simulink model "PR_planningsim_2joint"  (R2024a)
settings: Solver=ode45  StartTime=0.0  StopTime=stoptime
undefined symbols (not defined in the file): amp_factor, arm_radius, arm_radius_previus, begintime, controlactivate, damping_coeff, I_est, ifreskicking, ifreslosetrack, ifresnoise, ifrobotkicking, ifrobotnoise, ini_theta_p, ini_thetadot_p, pendepth, penlength, penposx, penposz, penrho, penwidth, rc, res_kick_height, res_kick_period, res_kick_start, res_losetrack_period, res_losetrack_start, res_noise_seed, res_noise_variance, robot_kick_height, robot_kick_period, robot_kick_start, robot_noise_seed, robot_noise_variance, robot_pendepth, robot_penlength, robot_penwidth, robot_pulse_freq, robot_pulse_hight, robot_pulse_period, robot_pulse_start, robot_sphere_mass, samplingrate, sphere_mass, sphere_radius, spring_position_scale, switch_threshold, torquelim, Win, X, Y, Z
libraries: sm_lib x25, nesl_utility x11, dspindex x5
(part 1 of 2)
settings Model: Creator=fy264  LastModifiedBy=fy264
settings OptimizationCC: ReuseModelBlockBuffer=off
settings DebuggingCC: AlgebraicLoopMsg=none  ArtificialAlgebraicLoopMsg=none
settings RTWCC: GPUComputeCapability=3.5
settings ExplorerConfigSet: InternalSimMechanicsExplorerSettings="<ExplorerConfiguration><canonicalview>default</canonicalview><AnimationSetting><BasePlaybackSpeed>1.0</BasePlaybackSpeed><PlaybackSpeedFactor>1.0</PlaybackSpeedFactor></AnimationSetting><TilePanel><TileInfo><Tiles Columns=\"1\" Count=\"1\" Rows=\"1\"><Column Weight=\"1\"/><Row Weight=\"1\"/><Tile Height=\"1\" Width=\"1\" X=\"0\" Y=\"0\"/></Tiles></TileInfo><SceneInfo><SceneViewer><BGColor><R>1</R><G>1</G><B>1</B></BGColor><Camera><DoPerspective>off</DoPerspective><Position><X>0.124591896750282635</X><Y>-1</Y><Z>0.0418966536850959165</Z></Position><Center><X>0.124591896750282635</X><Y>-3.46944695195361419e-18</Y><Z>0.0418966536850959165</Z></Center><Up><X>0</X><Y>-0</Y><Z>1</Z></Up><ViewLimDist>1</ViewLimDist><YLim>0.484627616003313111</YLim><XLim>0.343227538516062136</XLim></Camera></SceneViewer></SceneInfo></TilePanel><MechEditorPanel><Cameras/><GfxPanelCameraMap/><VideoCreator><PlaybackSpeedRatio>1.0</PlaybackSpeedRatio><FrameRate>30</FrameRate><VideoFormat>Motion JPEG AVI</VideoFormat><FrameSize>auto</FrameSize></VideoCreator></MechEditorPanel></ExplorerConfiguration>"

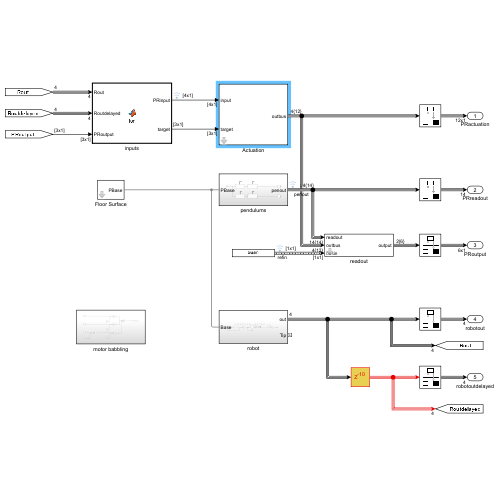
[thumbnail: Simulink's stored preview of the top-level diagram]
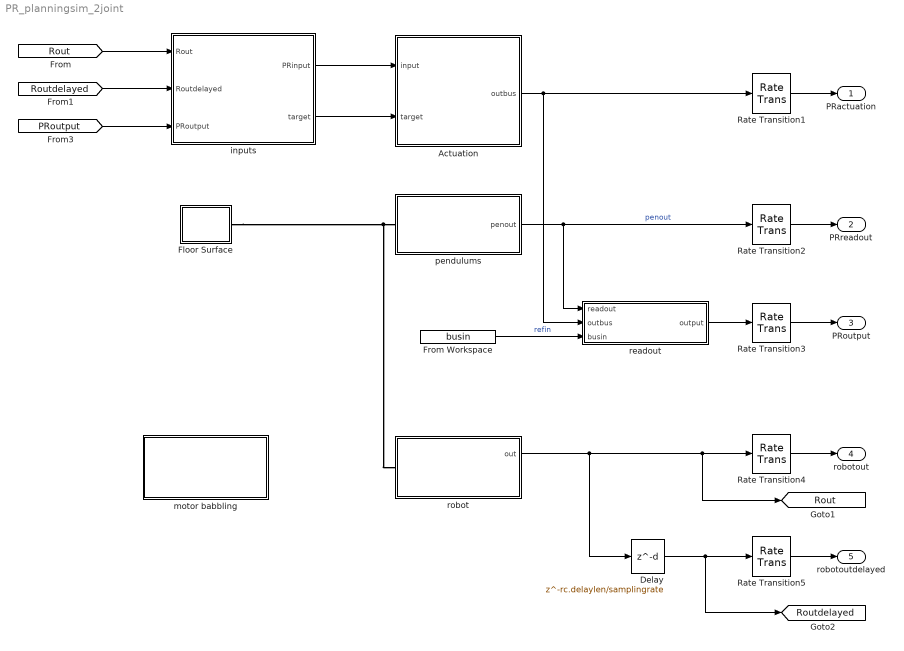
== system PR_planningsim_2joint ==
  Actuation : Subsystem  mask{xnorm=rc.xnorm}
  Delay : Delay  DelayLength=rc.delaylen/samplingrate  InitialCondition=0
  Floor Surface : Subsystem  mask{length=0.5, width=0.5}
      mask prompts: length "grid length [m]"; width "grid width [m]"
  From Workspace : FromWorkspace  VariableName=busin  OutDataTypeStr=Bus: SinusoidBus  OutputAfterFinalValue=Holding final value
  Rate Transition{1..5} (5 alike) : RateTransition  OutPortSampleTime=samplingrate
  inputs : MATLAB Function  TreatAsAtomicUnit=on
  motor babbling : Subsystem
  pendulums : Subsystem
  readout : Subsystem  mask{Woutmat=rc.Woutmat}
  robot : Subsystem
  PRactuation : Outport
  PRreadout : Outport  Port=2
  PRoutput : Outport  Port=3
  robotout : Outport  Port=4
  robotoutdelayed : Outport  Port=5
  tag scope: Rout=global, Routdelayed=global
  wires:
  Actuation/1(outbus) -> readout/2(outbus), Rate Transition1/1
  Rate Transition1/1 -> PRactuation/1
  pendulums/1(penout) -> readout/1(readout), Rate Transition2/1  "penout"
  Rate Transition2/1 -> PRreadout/1
  readout/1(output) -> Rate Transition3/1
  Rate Transition3/1 -> PRoutput/1
  Rate Transition4/1 -> robotout/1
  inputs/1(PRinput) -> Actuation/1(input)
  [Rout] -> inputs/1(Rout)
  Rate Transition5/1 -> robotoutdelayed/1
  robot/1(out) -> Delay/1, Rate Transition4/1, [Rout]
  Delay/1 -> [Routdelayed], Rate Transition5/1
  [Routdelayed] -> inputs/2(Routdelayed)
  inputs/2(target) -> Actuation/2(target)
  [PRoutput] -> inputs/3(PRoutput)
  From Workspace/1 -> readout/3(busin)  "refin"
  connections:
  Floor Surface/RConn1 -- robot/LConn1 -- pendulums/LConn1

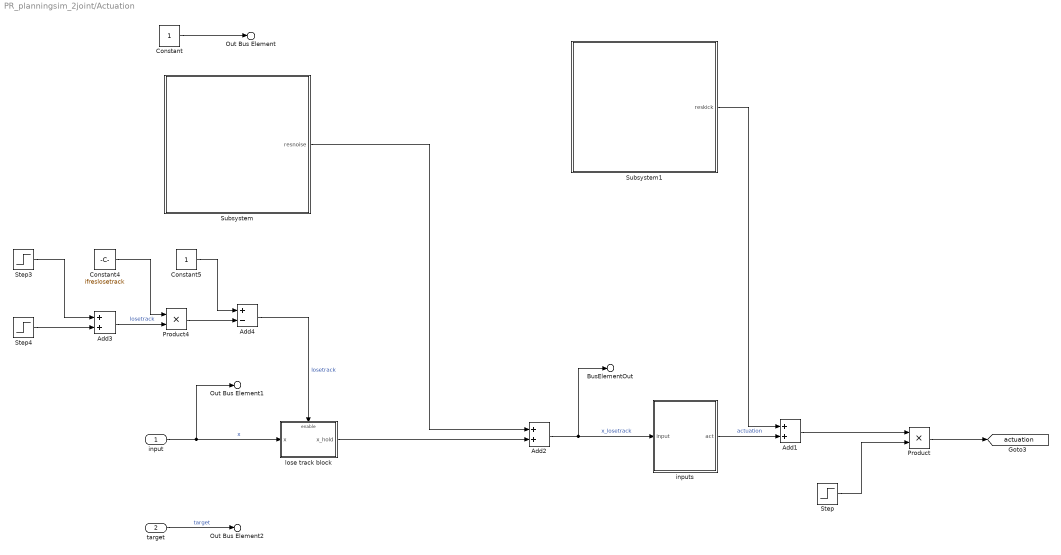
== system PR_planningsim_2joint/Actuation ==
  input : Inport
  target : Inport  Port=2
  Add1 : Sum
  Add2 : Sum
  Add3 : Sum
  Add4 : Sum  Inputs=+-
  Constant : Constant
  Constant4 : Constant  Value=ifreslosetrack
  Constant5 : Constant
  Product : Product
  Product4 : Product
  Step : Step  Time=begintime  SampleTime=0
  Step3 : Step  Time=res_losetrack_start  SampleTime=0
  Step4 : Step  Time=res_losetrack_start+res_losetrack_period  After=-1  SampleTime=0
  Subsystem : Subsystem
  Subsystem1 : Subsystem
  inputs : MATLAB Function  TreatAsAtomicUnit=on
  lose track block : Subsystem
  Out Bus Element : Outport  PortName=outbus  Element=const
  Out Bus Element1 : Outport  PortName=outbus  Element=x
  Out Bus Element2 : Outport  PortName=outbus  Element=target
  BusElementOut : Outport  PortName=outbus  Element=x_lost
  tag scope: actuation=global
  wires:
  input/1 -> Out Bus Element1/1, lose track block/1(x)  "x"
  Constant/1 -> Out Bus Element/1
  target/1 -> Out Bus Element2/1  "target"
  inputs/1(act) -> Add1/2  "actuation"
  Step/1 -> Product/2
  Step4/1 -> Add3/2
  Add3/1 -> Product4/2  "losetrack"
  Step3/1 -> Add3/1
  Constant4/1 -> Product4/1
  Constant5/1 -> Add4/1
  Product4/1 -> Add4/2
  Add4/1 -> lose track block/Enable  "losetrack"
  Product/1 -> [actuation]
  Add2/1 -> inputs/1(input), BusElementOut/1  "x_losetrack"
  Subsystem/1(resnoise) -> Add2/1
  lose track block/1(x_hold) -> Add2/2
  Add1/1 -> Product/1
  Subsystem1/1(reskick) -> Add1/1

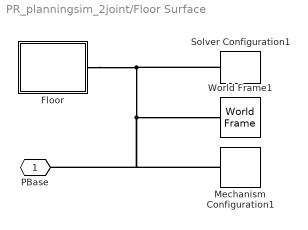
== system PR_planningsim_2joint/Floor Surface ==
  Floor : Subsystem
  Mechanism Configuration1 : sm_lib/Utilities/Mechanism Configuration  UniformGravity=Constant  GravityVector=[0 0 -9.80665]  GravityVectorUnits=m/s^2  LinearizationDelta=0.001  JointModeTransitionNonlinearIterations=2
  Solver Configuration1 : nesl_utility/Solver Configuration  PhysicalDomain=network_engine_domain  SubClassName=solver  LeftPortType=input  RightPortType=generic  Tones=[]  Harmonics=[]  SimulateNoise=off  Profile=off  UseLocalSampling=off  EnableSwitchedLinearOptims=on  FrequencyDomain=off  UseCCode=off  RelTol=0.001  AbsTol=1e-06  MinStep=1e-09  ToWorkspace=off  RevertToSquareIcSolve=off  NumHomotopyIterations=100  PhasorMode=off  PhasorModeNumHarmonics=1  ConsistencySolver=NEWTON_FTOL  IndexReductionMethod=DerivativeReplacement  DoDC=off  ResidualTolerance=1e-09  ConsistencyTolSource=GLOBAL  ConsistencyAbsTol=0.001  ConsistencyRelTol=0.001  ConsistencyTolFactor=0.001  UseLocalSolver=off  LocalSolverChoice=NE_BACKWARD_EULER_ADVANCER  ResolveIndetEquations=on  FunctionEvalNumThread=1  LocalSolverSampleTime=0.0002  DoFixedCost=off  MaxNonlinIter=10  MaxModeIter=2  ComputeImpulses=off  ImpulseIterations=2  LinearAlgebra=Sparse  LinearAlgebraNumThread=0  EquationFormulation=NE_TIME_EF  DelaysMemoryBudget=1024  AutomaticFiltering=off  FilteringTimeConstant=0.001  PartitionStorageMethod=AS_NEEDED  PartitionMemoryBudget=1024  PartitionMethod=FAST  MultibodyUseLocalSolver=off  MultibodyLocalSolverChoice=ODE1  MultibodyLocalSolverSampleTime=0.001
  World Frame1 : sm_lib/Frames and Transforms/World Frame
  PBase : PMIOPort  Side=Right
  connections:
  Floor/RConn1 -- PBase/RConn1 -- Mechanism Configuration1/RConn1 -- World Frame1/RConn1 -- Solver Configuration1/RConn1

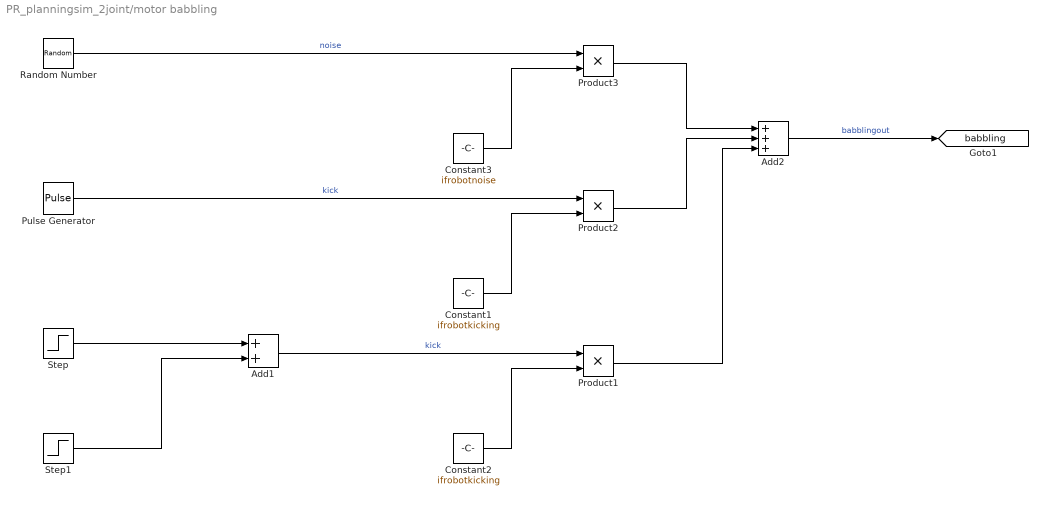
== system PR_planningsim_2joint/motor babbling ==
  Add1 : Sum
  Add2 : Sum  Inputs=+++
  Constant1 : Constant  Value=ifrobotkicking
  Constant2 : Constant  Value=ifrobotkicking
  Constant3 : Constant  Value=ifrobotnoise
  Product1 : Product
  Product2 : Product
  Product3 : Product
  Pulse Generator : DiscretePulseGenerator  PulseType=Time based  Amplitude=robot_pulse_hight  Period=1/robot_pulse_freq  PulseWidth=robot_pulse_period*robot_pulse_freq  PhaseDelay=robot_pulse_start
  Random Number : RandomNumber  Variance=robot_noise_variance  Seed=robot_noise_seed  SampleTime=samplingrate
  Step : Step  Time=robot_kick_start  After=robot_kick_height  SampleTime=0
  Step1 : Step  Time=robot_kick_start+robot_kick_period  After=-robot_kick_height  SampleTime=0
  tag scope: babbling=global
  wires:
  Step/1 -> Add1/1
  Step1/1 -> Add1/2
  Constant2/1 -> Product1/2
  Add2/1 -> [babbling]  "babblingout"
  Add1/1 -> Product1/1  "kick"
  Constant1/1 -> Product2/2
  Pulse Generator/1 -> Product2/1  "kick"
  Constant3/1 -> Product3/2
  Product3/1 -> Add2/1
  Product2/1 -> Add2/2
  Product1/1 -> Add2/3
  Random Number/1 -> Product3/1  "noise"

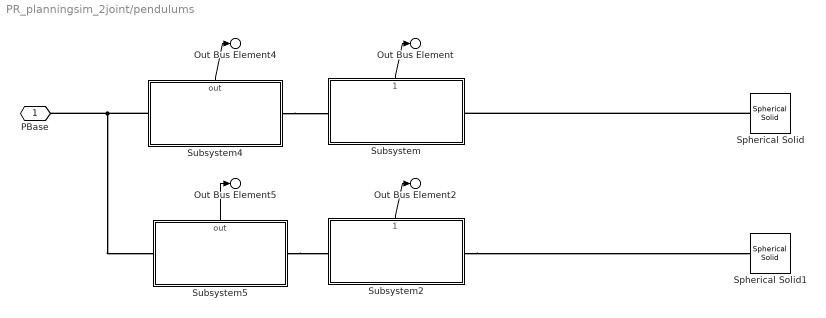
== system PR_planningsim_2joint/pendulums ==
  Spherical Solid : sm_lib/Body Elements/Spherical Solid  SphereRadius=sphere_radius(1, 3)  SphereRadiusUnits=m  ExportEntireGeometry=off  InertiaType=CalculateFromGeometry  BasedOnType=Mass  Density=1000  DensityUnits=kg/m^3  Mass=sphere_mass(1, 1)  MassUnits=kg  CenterOfMass=[0 0 0]  CenterOfMassUnits=m  MomentsOfInertia=[1 1 1]  MomentsOfInertiaUnits=kg*m^2  ProductsOfInertia=[0 0 0]  ProductsOfInertiaUnits=kg*m^2  GraphicType=FromGeometry  MarkerShape=Sphere  MarkerSize=10  GraphicVisPropType=SimpleVisualProperties  GraphicDiffuseColor=[0.6 0.6 0.6]  GraphicOpacity=1.0  GraphicSpecularColor=[0.5 0.5 0.5 1.0]  GraphicAmbientColor=[0.15 0.15 0.15 1.0]  GraphicEmissiveColor=[0.0 0.0 0.0 1.0]  GraphicShininess=75  DoExposeReferenceFrame=on  SerializedFrames=<Frames><Frame><Id>Frame1</Id><Value><Name>F1</Name><Origin><Source>ReferenceFrame</Source><FeatureName></FeatureName></Origin><PrimaryAxis><DefinedDirection>+Z</DefinedDirection><Source>ReferenceFrame</Source><SourceDirection>+Z</SourceDirection><FeatureName></FeatureName></PrimaryAxis><SecondaryAxis><DefinedDirection>+X</DefinedDirection><Source>ReferenceFrame</Source><SourceDirection>+X</SourceDirection><FeatureName></FeatureName></SecondaryAxis></Value></Frame></Frames>
  Spherical Solid1 : sm_lib/Body Elements/Spherical Solid  SphereRadius=sphere_radius(2, 3)  SphereRadiusUnits=m  ExportEntireGeometry=off  InertiaType=CalculateFromGeometry  BasedOnType=Mass  Density=1000  DensityUnits=kg/m^3  Mass=sphere_mass(1, 1)  MassUnits=kg  CenterOfMass=[0 0 0]  CenterOfMassUnits=m  MomentsOfInertia=[1 1 1]  MomentsOfInertiaUnits=kg*m^2  ProductsOfInertia=[0 0 0]  ProductsOfInertiaUnits=kg*m^2  GraphicType=FromGeometry  MarkerShape=Sphere  MarkerSize=10  GraphicVisPropType=SimpleVisualProperties  GraphicDiffuseColor=[0.6 0.6 0.6]  GraphicOpacity=1.0  GraphicSpecularColor=[0.5 0.5 0.5 1.0]  GraphicAmbientColor=[0.15 0.15 0.15 1.0]  GraphicEmissiveColor=[0.0 0.0 0.0 1.0]  GraphicShininess=75  DoExposeReferenceFrame=on  SerializedFrames=<Frames><Frame><Id>Frame1</Id><Value><Name>F1</Name><Origin><Source>ReferenceFrame</Source><FeatureName></FeatureName></Origin><PrimaryAxis><DefinedDirection>+Z</DefinedDirection><Source>ReferenceFrame</Source><SourceDirection>+Z</SourceDirection><FeatureName></FeatureName></PrimaryAxis><SecondaryAxis><DefinedDirection>+X</DefinedDirection><Source>ReferenceFrame</Source><SourceDirection>+X</SourceDirection><FeatureName></FeatureName></SecondaryAxis></Value></Frame></Frames>
  Subsystem : Subsystem  ReferencedSubsystem=pendulum_refsin  pendulum_label=[1 2]
      settings: PortSchema="{\"entries\":[{\"content\":{\"sides\":[{\"content\":{\"connectorIds\":[\"LConn1\"]},\"type\":\"ConnectorPlacement.EquallySpacedRectSide\",\"uuid\":\"2e961fb3-335c-4cac-865d-869b1ba40a20\"},{\"content\":{\"connectorIds\":[\"RConn1\"],\"side\":\"RIGHT\"},\"type\":\"ConnectorPlacement.EquallySpacedRectSide\",\"uuid\":\"69169429-8ae9-43d1-9e87-82c377e9f397\"},{\"content\":{\"connectorIds\":[\"Out1\"],\"side\":\"TOP\"},\"type\":\"ConnectorPlacement.EquallySpacedRectSide\",\"uuid\":\"d66a7b83-282b-4030-adef-01b228f0b3fc\"}]},\"type\":\"ConnectorPlacement.EquallySpacedConnector\",\"uuid\":\"3d306e9c-76f1-4223-9644-f2ea4df9a3d0\"}],\"packageUris\":[\"http://schema.mathworks.com/mf0/Connector/R2020b\"],\"version\":\"1.0\"}"
  Subsystem2 : Subsystem  ReferencedSubsystem=pendulum_refsin  pendulum_label=[2 2]
      settings: PortSchema="{\"entries\":[{\"content\":{\"sides\":[{\"content\":{\"connectorIds\":[\"LConn1\"]},\"type\":\"ConnectorPlacement.EquallySpacedRectSide\",\"uuid\":\"2e961fb3-335c-4cac-865d-869b1ba40a20\"},{\"content\":{\"connectorIds\":[\"RConn1\"],\"side\":\"RIGHT\"},\"type\":\"ConnectorPlacement.EquallySpacedRectSide\",\"uuid\":\"69169429-8ae9-43d1-9e87-82c377e9f397\"},{\"content\":{\"connectorIds\":[\"Out1\"],\"side\":\"TOP\"},\"type\":\"ConnectorPlacement.EquallySpacedRectSide\",\"uuid\":\"d66a7b83-282b-4030-adef-01b228f0b3fc\"}]},\"type\":\"ConnectorPlacement.EquallySpacedConnector\",\"uuid\":\"3d306e9c-76f1-4223-9644-f2ea4df9a3d0\"}],\"packageUris\":[\"http://schema.mathworks.com/mf0/Connector/R2020b\"],\"version\":\"1.0\"}"
  Subsystem4 : Subsystem  mask{pendulum_label=[1 1]}
      settings: PortSchema="{\"entries\":[{\"content\":{\"sides\":[{\"content\":{\"connectorIds\":[\"LConn1\"]},\"type\":\"ConnectorPlacement.EquallySpacedRectSide\",\"uuid\":\"2e961fb3-335c-4cac-865d-869b1ba40a20\"},{\"content\":{\"connectorIds\":[\"RConn1\"],\"side\":\"RIGHT\"},\"type\":\"ConnectorPlacement.EquallySpacedRectSide\",\"uuid\":\"69169429-8ae9-43d1-9e87-82c377e9f397\"},{\"content\":{\"connectorIds\":[\"Out1\"],\"side\":\"TOP\"},\"type\":\"ConnectorPlacement.EquallySpacedRectSide\",\"uuid\":\"d66a7b83-282b-4030-adef-01b228f0b3fc\"}]},\"type\":\"ConnectorPlacement.EquallySpacedConnector\",\"uuid\":\"3d306e9c-76f1-4223-9644-f2ea4df9a3d0\"}],\"packageUris\":[\"http://schema.mathworks.com/mf0/Connector/R2020b\"],\"version\":\"1.0\"}"
  Subsystem5 : Subsystem  mask{pendulum_label=[2 1]}
      settings: PortSchema="{\"entries\":[{\"content\":{\"sides\":[{\"content\":{\"connectorIds\":[\"LConn1\"]},\"type\":\"ConnectorPlacement.EquallySpacedRectSide\",\"uuid\":\"2e961fb3-335c-4cac-865d-869b1ba40a20\"},{\"content\":{\"connectorIds\":[\"RConn1\"],\"side\":\"RIGHT\"},\"type\":\"ConnectorPlacement.EquallySpacedRectSide\",\"uuid\":\"69169429-8ae9-43d1-9e87-82c377e9f397\"},{\"content\":{\"connectorIds\":[\"Out1\"],\"side\":\"TOP\"},\"type\":\"ConnectorPlacement.EquallySpacedRectSide\",\"uuid\":\"d66a7b83-282b-4030-adef-01b228f0b3fc\"}]},\"type\":\"ConnectorPlacement.EquallySpacedConnector\",\"uuid\":\"3d306e9c-76f1-4223-9644-f2ea4df9a3d0\"}],\"packageUris\":[\"http://schema.mathworks.com/mf0/Connector/R2020b\"],\"version\":\"1.0\"}"
  PBase : PMIOPort  Side=Left
  Out Bus Element4 : Outport  PortName=penout  Element=pendulum_1_0
  Out Bus Element : Outport  PortName=penout  Element=pendulum_1_1
  Out Bus Element5 : Outport  PortName=penout  Element=pendulum_2_0
  Out Bus Element2 : Outport  PortName=penout  Element=pendulum_2_1
  wires:
  Subsystem2/1 -> Out Bus Element2/1
  Subsystem/1 -> Out Bus Element/1
  Subsystem4/1(out) -> Out Bus Element4/1
  Subsystem5/1(out) -> Out Bus Element5/1
  connections:
  Spherical Solid/LConn1 -- Subsystem/RConn1
  Subsystem2/RConn1 -- Spherical Solid1/LConn1
  Subsystem4/RConn1 -- Subsystem/LConn1
  Subsystem4/LConn1 -- Subsystem5/LConn1 -- PBase/RConn1
  Subsystem5/RConn1 -- Subsystem2/LConn1

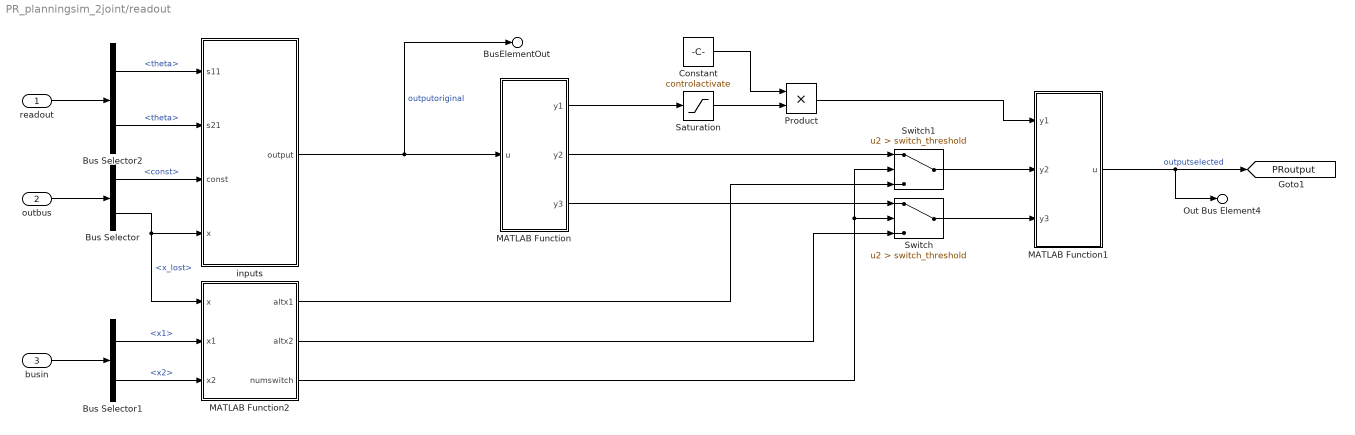
== system PR_planningsim_2joint/readout ==
  readout : Inport
  outbus : Inport  Port=2
  busin : Inport  Port=3
  Bus Selector : BusSelector  OutputSignals=const,x_lost
  Bus Selector1 : BusSelector  OutputSignals=x1,x2
  Bus Selector2 : BusSelector  OutputSignals=pendulum_1_1.theta,pendulum_2_1.theta
  Constant : Constant  Value=controlactivate
  MATLAB Function : MATLAB Function  TreatAsAtomicUnit=on
  MATLAB Function1 : MATLAB Function  TreatAsAtomicUnit=on
  MATLAB Function2 : MATLAB Function  TreatAsAtomicUnit=on
  Product : Product
  Saturation : Saturate  UpperLimit=torquelim  LowerLimit=-torquelim
  Switch : Switch  Criteria=u2 > Threshold  Threshold=switch_threshold  SaturateOnIntegerOverflow=off  InputSameDT=off
  Switch1 : Switch  Criteria=u2 > Threshold  Threshold=switch_threshold  SaturateOnIntegerOverflow=off  InputSameDT=off
  inputs : MATLAB Function  TreatAsAtomicUnit=on
  Out Bus Element4 : Outport  PortName=output  Element=outputselected
  BusElementOut : Outport  PortName=output  Element=outputoriginal
  tag scope: PRoutput=global
  wires:
  outbus/1 -> Bus Selector/1
  Bus Selector/1 -> inputs/3(const)  "<const>"
  Bus Selector/2 -> MATLAB Function2/1(x), inputs/4(x)  "<x_lost>"
  MATLAB Function1/1(u) -> Out Bus Element4/1, [PRoutput]  "outputselected"
  inputs/1(output) -> MATLAB Function/1(u), BusElementOut/1  "outputoriginal"
  MATLAB Function/1(y1) -> Saturation/1
  Saturation/1 -> Product/2
  Constant/1 -> Product/1
  busin/1 -> Bus Selector1/1
  MATLAB Function/2(y2) -> Switch1/1
  Switch1/1 -> MATLAB Function1/2(y2)
  Switch/1 -> MATLAB Function1/3(y3)
  Product/1 -> MATLAB Function1/1(y1)
  readout/1 -> Bus Selector2/1
  Bus Selector2/2 -> inputs/2(s21)  "<theta>"
  Bus Selector2/1 -> inputs/1(s11)  "<theta>"
  MATLAB Function/3(y3) -> Switch/1
  Bus Selector1/2 -> MATLAB Function2/3(x2)  "<x2>"
  Bus Selector1/1 -> MATLAB Function2/2(x1)  "<x1>"
  MATLAB Function2/1(altx1) -> Switch1/3
  MATLAB Function2/2(altx2) -> Switch/3
  MATLAB Function2/3(numswitch) -> Switch/2, Switch1/2

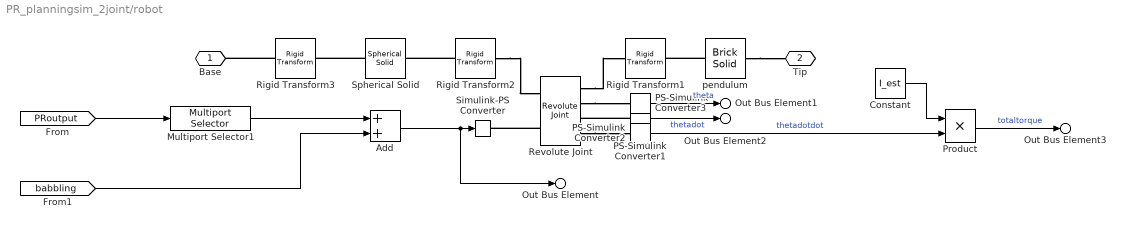
== system PR_planningsim_2joint/robot ==
  Add : Sum
  Constant : Constant  Value=I_est
  Multiport Selector1 : dspindex/Multiport Selector  rowsOrCols=Rows  idxCellArray=1  idxErrMode=Clip Index
  PS-Simulink Converter1 : nesl_utility/PS-Simulink Converter  PhysicalDomain=network_engine_domain  SubClassName=ps_output  LeftPortType=input  RightPortType=output  PseudoPeriodic=off  Frequencies=[]  VectorFormat=1-D array  Unit=1  AffineConversion=off
  PS-Simulink Converter2 : nesl_utility/PS-Simulink Converter  PhysicalDomain=network_engine_domain  SubClassName=ps_output  LeftPortType=input  RightPortType=output  PseudoPeriodic=off  Frequencies=[]  VectorFormat=1-D array  Unit=1  AffineConversion=off
  PS-Simulink Converter3 : nesl_utility/PS-Simulink Converter  PhysicalDomain=network_engine_domain  SubClassName=ps_output  LeftPortType=input  RightPortType=output  PseudoPeriodic=off  Frequencies=[]  VectorFormat=1-D array  Unit=1  AffineConversion=off
  Product : Product
  Revolute Joint : sm_lib/Joints/Revolute Joint  JointMode=Normal  CompositeWrenchDir=FollowerOnBase  CompositeWrenchFrame=BaseFrame  SenseConstraintForce=off  SenseConstraintTorque=off  SenseTotalForce=off  SenseTotalTorque=off  PositionTargetSpecify=on  PositionTargetPriority=Low  PositionTargetValue=robot_ini_theta_p  PositionTargetValueUnits=rad  VelocityTargetSpecify=on  VelocityTargetPriority=Low  VelocityTargetValue=robot_ini_thetadot_p  VelocityTargetValueUnits=rad/s  EquilibriumPosition=0  EquilibriumPositionUnits=rad  SpringStiffness=0  SpringStiffnessUnits=N*m/rad  DampingCoefficient=robot_damping_coeff  DampingCoefficientUnits=N*m/(rad/s)  LowerLimitSpecify=off  LowerLimitBound=-90  LowerLimitBoundUnits=deg  LowerLimitStiffness=1e4  LowerLimitStiffnessUnits=N*m/deg  LowerLimitDamping=10  LowerLimitDampingUnits=N*m/(deg/s)  LowerLimitTransitionRegionWidth=0.1  LowerLimitTransitionRegionWidthUnits=deg  UpperLimitSpecify=off  UpperLimitBound=90  UpperLimitBoundUnits=deg  UpperLimitStiffness=1e4  UpperLimitStiffnessUnits=N*m/deg  UpperLimitDamping=10  UpperLimitDampingUnits=N*m/(deg/s)  UpperLimitTransitionRegionWidth=0.1  UpperLimitTransitionRegionWidthUnits=deg  TorqueActuationMode=InputTorque  MotionActuationMode=ComputedMotion  SensePosition=on  SenseVelocity=on  SenseAcceleration=on  SenseTorqueForce=off  SenseLowerLimitTorqueForce=off  SenseUpperLimitTorqueForce=off
  Rigid Transform1 : sm_lib/Frames and Transforms/Rigid Transform  RotationMethod=AlignedAxes  FollAlignAxisA=+X  BaseAlignAxisA=+X  FollAlignAxisB=-Z  BaseAlignAxisB=+Y  RotationStandardAxis=+Z  RotationAngle=180  RotationAngleUnits=deg  RotationArbitraryAxis=[0 0 1]  RotationSequenceAxes=FollowerAxes  RotationSequence=XYX  RotationSequenceAngles=[0 0 0]  RotationSequenceAnglesUnits=deg  RotationMatrix=[1 0 0; 0 1 0; 0 0 1]  Quaternion=[1 0 0 0]  TranslationMethod=None  TranslationCartesianOffset=[arm_radius*spring_position_scale 0 0]  TranslationCartesianOffsetUnits=m  TranslationStandardAxis=+Z  TranslationStandardOffset=0  TranslationStandardOffsetUnits=m  TranslationROffset=arm_radius_previus*spring_position_scale  TranslationROffsetUnits=m  TranslationThetaOffset=theta  TranslationThetaOffsetUnits=deg  TranslationZOffset=0  TranslationZOffsetUnits=m
  Rigid Transform2 : sm_lib/Frames and Transforms/Rigid Transform  RotationMethod=AlignedAxes  FollAlignAxisA=+X  BaseAlignAxisA=+X  FollAlignAxisB=+Y  BaseAlignAxisB=+Z  RotationStandardAxis=+Z  RotationAngle=180  RotationAngleUnits=deg  RotationArbitraryAxis=[0 0 1]  RotationSequenceAxes=FollowerAxes  RotationSequence=XYX  RotationSequenceAngles=[0 0 0]  RotationSequenceAnglesUnits=deg  RotationMatrix=[1 0 0; 0 1 0; 0 0 1]  Quaternion=[1 0 0 0]  TranslationMethod=None  TranslationCartesianOffset=[arm_radius*spring_position_scale 0 0]  TranslationCartesianOffsetUnits=m  TranslationStandardAxis=+Z  TranslationStandardOffset=0  TranslationStandardOffsetUnits=m  TranslationROffset=arm_radius_previus*spring_position_scale  TranslationROffsetUnits=m  TranslationThetaOffset=theta  TranslationThetaOffsetUnits=deg  TranslationZOffset=0  TranslationZOffsetUnits=m
  Rigid Transform3 : sm_lib/Frames and Transforms/Rigid Transform  RotationMethod=None  FollAlignAxisA=+X  BaseAlignAxisA=+X  FollAlignAxisB=+Y  BaseAlignAxisB=+Z  RotationStandardAxis=+Z  RotationAngle=180  RotationAngleUnits=deg  RotationArbitraryAxis=[0 0 1]  RotationSequenceAxes=FollowerAxes  RotationSequence=XYX  RotationSequenceAngles=[0 0 0]  RotationSequenceAnglesUnits=deg  RotationMatrix=[1 0 0; 0 1 0; 0 0 1]  Quaternion=[1 0 0 0]  TranslationMethod=StandardAxis  TranslationCartesianOffset=[arm_radius*spring_position_scale 0 0]  TranslationCartesianOffsetUnits=m  TranslationStandardAxis=+Z  TranslationStandardOffset=robot_penposz  TranslationStandardOffsetUnits=m  TranslationROffset=arm_radius_previus*spring_position_scale  TranslationROffsetUnits=m  TranslationThetaOffset=theta  TranslationThetaOffsetUnits=deg  TranslationZOffset=0  TranslationZOffsetUnits=m
  Simulink-PS Converter : nesl_utility/Simulink-PS Converter  PhysicalDomain=network_engine_domain  SubClassName=ps_input  LeftPortType=input  RightPortType=output  PseudoPeriodic=off  Frequencies=[]  NoiseDistribution=none  NoiseParameters=[]  Unit=1  AffineConversion=off  FilteringAndDerivatives=provide  SimscapeFilterOrder=1  InputFilterTimeConstant=0.001  UdotUserProvided=0
  Spherical Solid : sm_lib/Body Elements/Spherical Solid  SphereRadius=robot_sphere_radius  SphereRadiusUnits=m  ExportEntireGeometry=off  InertiaType=CalculateFromGeometry  BasedOnType=Mass  Density=1000  DensityUnits=kg/m^3  Mass=robot_sphere_mass  MassUnits=kg  CenterOfMass=[0 0 0]  CenterOfMassUnits=m  MomentsOfInertia=[1 1 1]  MomentsOfInertiaUnits=kg*m^2  ProductsOfInertia=[0 0 0]  ProductsOfInertiaUnits=kg*m^2  GraphicType=FromGeometry  MarkerShape=Sphere  MarkerSize=10  GraphicVisPropType=SimpleVisualProperties  GraphicDiffuseColor=[0.6 0.6 0.6]  GraphicOpacity=1.0  GraphicSpecularColor=[0.5 0.5 0.5 1.0]  GraphicAmbientColor=[0.15 0.15 0.15 1.0]  GraphicEmissiveColor=[0.0 0.0 0.0 1.0]  GraphicShininess=75  DoExposeReferenceFrame=on  SerializedFrames=<Frames><Frame><Id>Frame1</Id><Value><Name>F1</Name><Origin><Source>ReferenceFrame</Source><FeatureName></FeatureName></Origin><PrimaryAxis><DefinedDirection>+Z</DefinedDirection><Source>ReferenceFrame</Source><SourceDirection>+Z</SourceDirection><FeatureName></FeatureName></PrimaryAxis><SecondaryAxis><DefinedDirection>+X</DefinedDirection><Source>ReferenceFrame</Source><SourceDirection>+X</SourceDirection><FeatureName></FeatureName></SecondaryAxis></Value></Frame></Frames>
  pendulum : sm_lib/Body Elements/Brick Solid  BrickDimensions=[robot_penwidth robot_pendepth robot_penlength]  BrickDimensionsUnits=m  ExportEntireGeometry=off  InertiaType=CalculateFromGeometry  BasedOnType=Density  Density=robot_penrho  DensityUnits=kg/m^3  Mass=1  MassUnits=kg  CenterOfMass=[0 0 0]  CenterOfMassUnits=m  MomentsOfInertia=[1 1 1]  MomentsOfInertiaUnits=kg*m^2  ProductsOfInertia=[0 0 0]  ProductsOfInertiaUnits=kg*m^2  GraphicType=FromGeometry  MarkerShape=Sphere  MarkerSize=10  GraphicVisPropType=SimpleVisualProperties  GraphicDiffuseColor=[0.0 0.0 1.0]  GraphicOpacity=1.0  GraphicSpecularColor=[0.5 0.5 0.5 1.0]  GraphicAmbientColor=[0.15 0.15 0.15 1.0]  GraphicEmissiveColor=[0.0 0.0 0.0 1.0]  GraphicShininess=75  DoExposeReferenceFrame=off  SerializedFrames=<Frames><Frame><Id>Frame1</Id><Value><Name>F1</Name><Origin><Source>GeometricFeature</Source><FeatureName>-z surface</FeatureName></Origin><PrimaryAxis><DefinedDirection>+Z</DefinedDirection><Source>ReferenceFrame</Source><SourceDirection>+Z</SourceDirection><FeatureName></FeatureName></PrimaryAxis><SecondaryAxis><DefinedDirection>+X</DefinedDirection><Source>ReferenceFrame</Source><SourceDirection>+X</SourceDirection><FeatureName></FeatureName></SecondaryAxis></Value></Frame><Frame><Id>Frame2</Id><Value><Name>F2</Name><Origin><Source>GeometricFeature</Source><FeatureName>+z surface</FeatureName></Origin><PrimaryAxis><DefinedDirection>+Z</DefinedDirection><Source>ReferenceFrame</Source><SourceDirection>-Z</SourceDirection><FeatureName></FeatureName></PrimaryAxis><SecondaryAxis><DefinedDirection>+X</DefinedDirection><Source>ReferenceFrame</Source><SourceDirection>+X</SourceDirection><FeatureName></FeatureName></SecondaryAxis></Value></Frame></Frames>
  Base : PMIOPort  Side=Left
  Tip : PMIOPort  Port=2  Side=Right
  Out Bus Element1 : Outport  PortName=out  Element=theta
  Out Bus Element2 : Outport  PortName=out  Element=thetadot
  Out Bus Element3 : Outport  PortName=out  Element=totaltorque
  Out Bus Element : Outport  PortName=out  Element=actuationtorque
  wires:
  PS-Simulink Converter3/1 -> Out Bus Element1/1  "theta"
  PS-Simulink Converter1/1 -> Out Bus Element2/1  "thetadot"
  PS-Simulink Converter2/1 -> Product/2  "thetadotdot"
  Product/1 -> Out Bus Element3/1  "totaltorque"
  Constant/1 -> Product/1
  [PRoutput] -> Multiport Selector1/1
  Multiport Selector1/1 -> Add/1
  [babbling] -> Add/2
  Add/1 -> Out Bus Element/1, Simulink-PS Converter/1
  connections:
  Revolute Joint/LConn2 -- Simulink-PS Converter/RConn1
  Revolute Joint/RConn2 -- PS-Simulink Converter3/LConn1
  Rigid Transform2/LConn1 -- Spherical Solid/RConn1
  PS-Simulink Converter1/LConn1 -- Revolute Joint/RConn3
  Spherical Solid/LConn1 -- Rigid Transform3/RConn1
  pendulum/LConn1 -- Rigid Transform1/RConn1
  Rigid Transform3/LConn1 -- Base/RConn1
  pendulum/RConn1 -- Tip/RConn1
  Rigid Transform2/RConn1 -- Revolute Joint/LConn1
  Revolute Joint/RConn4 -- PS-Simulink Converter2/LConn1
  Revolute Joint/RConn1 -- Rigid Transform1/LConn1

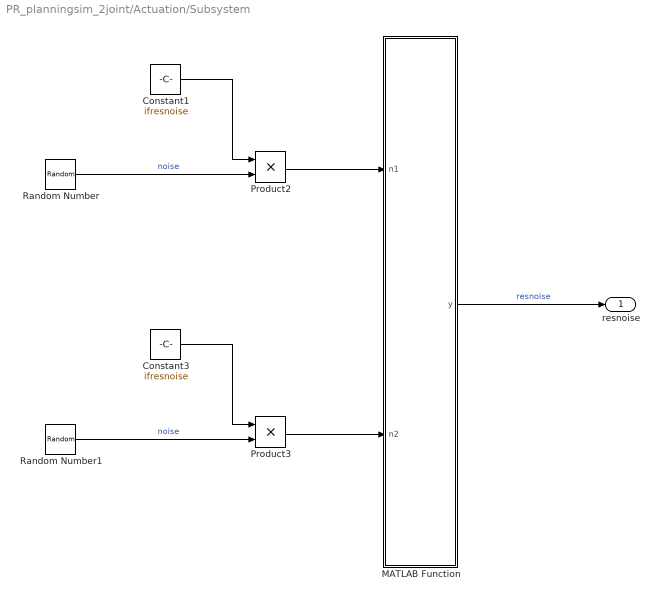
== system PR_planningsim_2joint/Actuation/Subsystem ==
  Constant1 : Constant  Value=ifresnoise
  Constant3 : Constant  Value=ifresnoise
  MATLAB Function : MATLAB Function  TreatAsAtomicUnit=on
  Product2 : Product
  Product3 : Product
  Random Number : RandomNumber  Variance=res_noise_variance(1)  Seed=res_noise_seed(1)  SampleTime=samplingrate
  Random Number1 : RandomNumber  Variance=res_noise_variance(2)  Seed=res_noise_seed(2)  SampleTime=samplingrate
  resnoise : Outport
  wires:
  MATLAB Function/1(y) -> resnoise/1  "resnoise"
  Constant3/1 -> Product3/1
  Product2/1 -> MATLAB Function/1(n1)
  Random Number1/1 -> Product3/2  "noise"
  Product3/1 -> MATLAB Function/2(n2)
  Constant1/1 -> Product2/1
  Random Number/1 -> Product2/2  "noise"

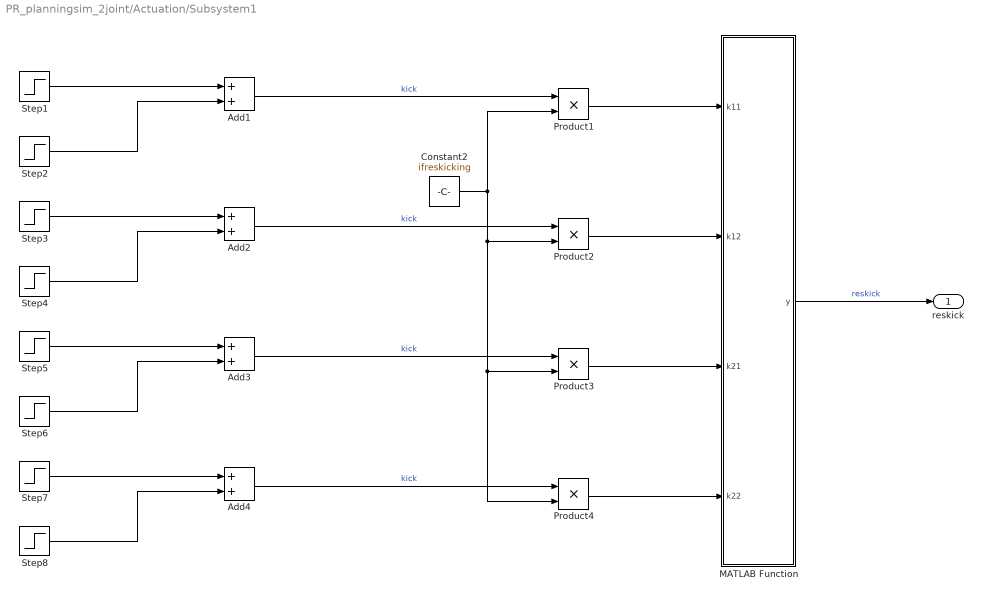
== system PR_planningsim_2joint/Actuation/Subsystem1 ==
  Add{1..4} (4 alike) : Sum
  Constant2 : Constant  Value=ifreskicking
  MATLAB Function : MATLAB Function  TreatAsAtomicUnit=on
  Product{1..4} (4 alike) : Product
  Step1 : Step  Time=res_kick_start(1,1)  After=res_kick_height(1,1)  SampleTime=0
  Step2 : Step  Time=res_kick_start(1,1)+res_kick_period(1,1)  After=-res_kick_height(1,1)  SampleTime=0
  Step3 : Step  Time=res_kick_start(1,2)  After=res_kick_height(1,2)  SampleTime=0
  Step4 : Step  Time=res_kick_start(1,2)+res_kick_period(1,2)  After=-res_kick_height(1,2)  SampleTime=0
  Step5 : Step  Time=res_kick_start(2,1)  After=res_kick_height(2,1)  SampleTime=0
  Step6 : Step  Time=res_kick_start(2,1)+res_kick_period(2,1)  After=-res_kick_height(2,1)  SampleTime=0
  Step7 : Step  Time=res_kick_start(2,2)  After=res_kick_height(2,2)  SampleTime=0
  Step8 : Step  Time=res_kick_start(2,2)+res_kick_period(2,2)  After=-res_kick_height(2,2)  SampleTime=0
  reskick : Outport
  wires:
  Add1/1 -> Product1/1  "kick"
  Step2/1 -> Add1/2
  Step1/1 -> Add1/1
  MATLAB Function/1(y) -> reskick/1  "reskick"
  Product1/1 -> MATLAB Function/1(k11)
  Step4/1 -> Add2/2
  Add2/1 -> Product2/1  "kick"
  Step3/1 -> Add2/1
  Product2/1 -> MATLAB Function/2(k12)
  Step6/1 -> Add3/2
  Add3/1 -> Product3/1  "kick"
  Step5/1 -> Add3/1
  Product3/1 -> MATLAB Function/3(k21)
  Step8/1 -> Add4/2
  Step7/1 -> Add4/1
  Add4/1 -> Product4/1  "kick"
  Constant2/1 -> Product4/2, Product3/2, Product2/2, Product1/2
  Product4/1 -> MATLAB Function/4(k22)

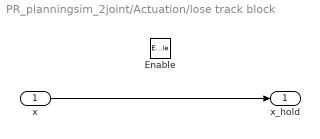
== system PR_planningsim_2joint/Actuation/lose track block ==
  x : Inport
  Enable : EnablePort
  x_hold : Outport
  wires:
  x/1 -> x_hold/1

== system PR_planningsim_2joint/Floor Surface/Floor ==
  Grid : Subsystem  mask(Grid Lines){grid_origin=[-length -width 0], grid_size=[length width], grid_linewidth=0.001, grid_num_squares=20, grid_color=[0.8 0.8 0.8], grid_opacity=0.8}
      mask prompts: grid_origin "Origin (m)"; grid_size "Arena size (m)"; grid_linewidth "Grid Line Width (m)"; grid_num_squares "Number of Squares"; grid_color "Grid Color [RGB]"; grid_opacity "Grid Opacity (0-1)"
      mask help: Creates grids on 3 planes XZ, YZ, and XZ.
      mask init:
      | mesh_xsec = Extr_Data_Mesh(grid_size(1), grid_size(2), grid_num_squares, grid_num_squares, grid_size(1)/grid_num_squares-grid_linewidth, grid_size(2)/grid_num_squares-grid_linewidth);
  Ref : PMIOPort  Side=Right
  connections:
  Grid/LConn1 -- Ref/RConn1

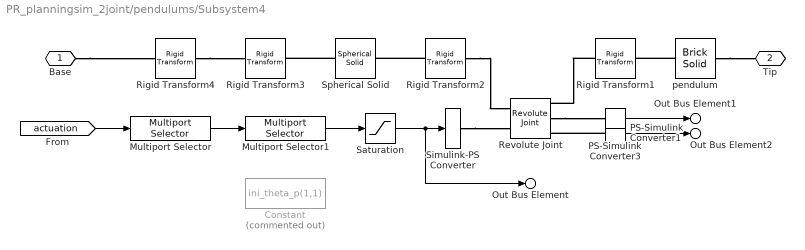
== system PR_planningsim_2joint/pendulums/Subsystem4 ==
  Constant : Constant  Commented=on  Value=ini_theta_p(1,1)
  Multiport Selector : dspindex/Multiport Selector  rowsOrCols=Rows  idxCellArray=pendulum_label(1)  idxErrMode=Clip Index
  Multiport Selector1 : dspindex/Multiport Selector  rowsOrCols=Columns  idxCellArray=pendulum_label(2)  idxErrMode=Clip Index
  PS-Simulink Converter1 : nesl_utility/PS-Simulink Converter  PhysicalDomain=network_engine_domain  SubClassName=ps_output  LeftPortType=input  RightPortType=output  PseudoPeriodic=off  Frequencies=[]  VectorFormat=1-D array  Unit=1  AffineConversion=off
  PS-Simulink Converter3 : nesl_utility/PS-Simulink Converter  PhysicalDomain=network_engine_domain  SubClassName=ps_output  LeftPortType=input  RightPortType=output  PseudoPeriodic=off  Frequencies=[]  VectorFormat=1-D array  Unit=1  AffineConversion=off
  Revolute Joint : sm_lib/Joints/Revolute Joint  JointMode=Normal  CompositeWrenchDir=FollowerOnBase  CompositeWrenchFrame=BaseFrame  SenseConstraintForce=off  SenseConstraintTorque=off  SenseTotalForce=off  SenseTotalTorque=off  PositionTargetSpecify=on  PositionTargetPriority=High  PositionTargetValue=ini_theta_p(pendulum_label(1), pendulum_label(2))  PositionTargetValueUnits=rad  VelocityTargetSpecify=on  VelocityTargetPriority=High  VelocityTargetValue=ini_thetadot_p(pendulum_label(1), pendulum_label(2))  VelocityTargetValueUnits=rad/s  EquilibriumPosition=0  EquilibriumPositionUnits=rad  SpringStiffness=0  SpringStiffnessUnits=N*m/rad  DampingCoefficient=damping_coeff(pendulum_label(1), pendulum_label(2))  DampingCoefficientUnits=N*m/(rad/s)  LowerLimitSpecify=off  LowerLimitBound=-90  LowerLimitBoundUnits=deg  LowerLimitStiffness=1e4  LowerLimitStiffnessUnits=N*m/deg  LowerLimitDamping=10  LowerLimitDampingUnits=N*m/(deg/s)  LowerLimitTransitionRegionWidth=0.1  LowerLimitTransitionRegionWidthUnits=deg  UpperLimitSpecify=off  UpperLimitBound=90  UpperLimitBoundUnits=deg  UpperLimitStiffness=1e4  UpperLimitStiffnessUnits=N*m/deg  UpperLimitDamping=10  UpperLimitDampingUnits=N*m/(deg/s)  UpperLimitTransitionRegionWidth=0.1  UpperLimitTransitionRegionWidthUnits=deg  TorqueActuationMode=ComputedTorque  MotionActuationMode=InputMotion  SensePosition=on  SenseVelocity=on  SenseAcceleration=off  SenseTorqueForce=off  SenseLowerLimitTorqueForce=off  SenseUpperLimitTorqueForce=off
  Rigid Transform1 : sm_lib/Frames and Transforms/Rigid Transform  RotationMethod=AlignedAxes  FollAlignAxisA=+X  BaseAlignAxisA=+X  FollAlignAxisB=-Z  BaseAlignAxisB=+Y  RotationStandardAxis=+Z  RotationAngle=180  RotationAngleUnits=deg  RotationArbitraryAxis=[0 0 1]  RotationSequenceAxes=FollowerAxes  RotationSequence=XYX  RotationSequenceAngles=[0 0 0]  RotationSequenceAnglesUnits=deg  RotationMatrix=[1 0 0; 0 1 0; 0 0 1]  Quaternion=[1 0 0 0]  TranslationMethod=None  TranslationCartesianOffset=[arm_radius*spring_position_scale 0 0]  TranslationCartesianOffsetUnits=m  TranslationStandardAxis=+Z  TranslationStandardOffset=0  TranslationStandardOffsetUnits=m  TranslationROffset=arm_radius_previus*spring_position_scale  TranslationROffsetUnits=m  TranslationThetaOffset=theta  TranslationThetaOffsetUnits=deg  TranslationZOffset=0  TranslationZOffsetUnits=m
  Rigid Transform2 : sm_lib/Frames and Transforms/Rigid Transform  RotationMethod=AlignedAxes  FollAlignAxisA=+X  BaseAlignAxisA=+X  FollAlignAxisB=+Y  BaseAlignAxisB=+Z  RotationStandardAxis=+Z  RotationAngle=180  RotationAngleUnits=deg  RotationArbitraryAxis=[0 0 1]  RotationSequenceAxes=FollowerAxes  RotationSequence=XYX  RotationSequenceAngles=[0 0 0]  RotationSequenceAnglesUnits=deg  RotationMatrix=[1 0 0; 0 1 0; 0 0 1]  Quaternion=[1 0 0 0]  TranslationMethod=None  TranslationCartesianOffset=[arm_radius*spring_position_scale 0 0]  TranslationCartesianOffsetUnits=m  TranslationStandardAxis=+Z  TranslationStandardOffset=0  TranslationStandardOffsetUnits=m  TranslationROffset=arm_radius_previus*spring_position_scale  TranslationROffsetUnits=m  TranslationThetaOffset=theta  TranslationThetaOffsetUnits=deg  TranslationZOffset=0  TranslationZOffsetUnits=m
  Rigid Transform3 : sm_lib/Frames and Transforms/Rigid Transform  RotationMethod=None  FollAlignAxisA=+X  BaseAlignAxisA=+X  FollAlignAxisB=+Y  BaseAlignAxisB=+Z  RotationStandardAxis=+Z  RotationAngle=180  RotationAngleUnits=deg  RotationArbitraryAxis=[0 0 1]  RotationSequenceAxes=FollowerAxes  RotationSequence=XYX  RotationSequenceAngles=[0 0 0]  RotationSequenceAnglesUnits=deg  RotationMatrix=[1 0 0; 0 1 0; 0 0 1]  Quaternion=[1 0 0 0]  TranslationMethod=StandardAxis  TranslationCartesianOffset=[arm_radius*spring_position_scale 0 0]  TranslationCartesianOffsetUnits=m  TranslationStandardAxis=+X  TranslationStandardOffset=penposx(pendulum_label(1), pendulum_label(2))  TranslationStandardOffsetUnits=m  TranslationROffset=arm_radius_previus*spring_position_scale  TranslationROffsetUnits=m  TranslationThetaOffset=theta  TranslationThetaOffsetUnits=deg  TranslationZOffset=0  TranslationZOffsetUnits=m
  Rigid Transform4 : sm_lib/Frames and Transforms/Rigid Transform  RotationMethod=None  FollAlignAxisA=+X  BaseAlignAxisA=+X  FollAlignAxisB=+Y  BaseAlignAxisB=+Z  RotationStandardAxis=+Z  RotationAngle=180  RotationAngleUnits=deg  RotationArbitraryAxis=[0 0 1]  RotationSequenceAxes=FollowerAxes  RotationSequence=XYX  RotationSequenceAngles=[0 0 0]  RotationSequenceAnglesUnits=deg  RotationMatrix=[1 0 0; 0 1 0; 0 0 1]  Quaternion=[1 0 0 0]  TranslationMethod=StandardAxis  TranslationCartesianOffset=[arm_radius*spring_position_scale 0 0]  TranslationCartesianOffsetUnits=m  TranslationStandardAxis=+Z  TranslationStandardOffset=penposz(pendulum_label(1), pendulum_label(2))  TranslationStandardOffsetUnits=m  TranslationROffset=arm_radius_previus*spring_position_scale  TranslationROffsetUnits=m  TranslationThetaOffset=theta  TranslationThetaOffsetUnits=deg  TranslationZOffset=0  TranslationZOffsetUnits=m
  Saturation : Saturate  UpperLimit=pi/2  LowerLimit=-pi/2
  Simulink-PS Converter : nesl_utility/Simulink-PS Converter  PhysicalDomain=network_engine_domain  SubClassName=ps_input  LeftPortType=input  RightPortType=output  PseudoPeriodic=off  Frequencies=[]  NoiseDistribution=none  NoiseParameters=[]  Unit=1  AffineConversion=off  FilteringAndDerivatives=filter  SimscapeFilterOrder=2  InputFilterTimeConstant=0.05  UdotUserProvided=0
  Spherical Solid : sm_lib/Body Elements/Spherical Solid  SphereRadius=sphere_radius(pendulum_label(1), pendulum_label(2))  SphereRadiusUnits=m  ExportEntireGeometry=off  InertiaType=CalculateFromGeometry  BasedOnType=Mass  Density=1000  DensityUnits=kg/m^3  Mass=sphere_mass(pendulum_label(1), pendulum_label(2))  MassUnits=kg  CenterOfMass=[0 0 0]  CenterOfMassUnits=m  MomentsOfInertia=[1 1 1]  MomentsOfInertiaUnits=kg*m^2  ProductsOfInertia=[0 0 0]  ProductsOfInertiaUnits=kg*m^2  GraphicType=FromGeometry  MarkerShape=Sphere  MarkerSize=10  GraphicVisPropType=SimpleVisualProperties  GraphicDiffuseColor=[0.6 0.6 0.6]  GraphicOpacity=1.0  GraphicSpecularColor=[0.5 0.5 0.5 1.0]  GraphicAmbientColor=[0.15 0.15 0.15 1.0]  GraphicEmissiveColor=[0.0 0.0 0.0 1.0]  GraphicShininess=75  DoExposeReferenceFrame=on  SerializedFrames=<Frames><Frame><Id>Frame1</Id><Value><Name>F1</Name><Origin><Source>ReferenceFrame</Source><FeatureName></FeatureName></Origin><PrimaryAxis><DefinedDirection>+Z</DefinedDirection><Source>ReferenceFrame</Source><SourceDirection>+Z</SourceDirection><FeatureName></FeatureName></PrimaryAxis><SecondaryAxis><DefinedDirection>+X</DefinedDirection><Source>ReferenceFrame</Source><SourceDirection>+X</SourceDirection><FeatureName></FeatureName></SecondaryAxis></Value></Frame></Frames>
  pendulum : sm_lib/Body Elements/Brick Solid  BrickDimensions=[penwidth(pendulum_label(1), pendulum_label(2)) pendepth(pendulum_label(1), pendulum_label(2)) penlength(pendulum_label(1), pendulum_label(2))]  BrickDimensionsUnits=m  ExportEntireGeometry=off  InertiaType=CalculateFromGeometry  BasedOnType=Density  Density=penrho(pendulum_label(1), pendulum_label(2))  DensityUnits=kg/m^3  Mass=1  MassUnits=kg  CenterOfMass=[0 0 0]  CenterOfMassUnits=m  MomentsOfInertia=[1 1 1]  MomentsOfInertiaUnits=kg*m^2  ProductsOfInertia=[0 0 0]  ProductsOfInertiaUnits=kg*m^2  GraphicType=FromGeometry  MarkerShape=Sphere  MarkerSize=10  GraphicVisPropType=SimpleVisualProperties  GraphicDiffuseColor=[1.0 0.0 0.0]  GraphicOpacity=1.0  GraphicSpecularColor=[0.5 0.5 0.5 1.0]  GraphicAmbientColor=[0.15 0.15 0.15 1.0]  GraphicEmissiveColor=[0.0 0.0 0.0 1.0]  GraphicShininess=75  DoExposeReferenceFrame=off  SerializedFrames=<Frames><Frame><Id>Frame1</Id><Value><Name>F1</Name><Origin><Source>GeometricFeature</Source><FeatureName>-z surface</FeatureName></Origin><PrimaryAxis><DefinedDirection>+Z</DefinedDirection><Source>ReferenceFrame</Source><SourceDirection>+Z</SourceDirection><FeatureName></FeatureName></PrimaryAxis><SecondaryAxis><DefinedDirection>+X</DefinedDirection><Source>ReferenceFrame</Source><SourceDirection>+X</SourceDirection><FeatureName></FeatureName></SecondaryAxis></Value></Frame><Frame><Id>Frame2</Id><Value><Name>F2</Name><Origin><Source>GeometricFeature</Source><FeatureName>+z surface</FeatureName></Origin><PrimaryAxis><DefinedDirection>+Z</DefinedDirection><Source>ReferenceFrame</Source><SourceDirection>-Z</SourceDirection><FeatureName></FeatureName></PrimaryAxis><SecondaryAxis><DefinedDirection>+X</DefinedDirection><Source>ReferenceFrame</Source><SourceDirection>+X</SourceDirection><FeatureName></FeatureName></SecondaryAxis></Value></Frame></Frames>
  Base : PMIOPort  Side=Left
  Tip : PMIOPort  Port=2  Side=Right
  Out Bus Element : Outport  PortName=out  Element=torque
  Out Bus Element1 : Outport  PortName=out  Element=theta
  Out Bus Element2 : Outport  PortName=out  Element=thetadot
  wires:
  PS-Simulink Converter3/1 -> Out Bus Element1/1
  PS-Simulink Converter1/1 -> Out Bus Element2/1
  Multiport Selector/1 -> Multiport Selector1/1
  Saturation/1 -> Simulink-PS Converter/1, Out Bus Element/1
  [actuation] -> Multiport Selector/1
  Multiport Selector1/1 -> Saturation/1
  connections:
  Spherical Solid/LConn1 -- Rigid Transform3/RConn1
  Rigid Transform1/LConn1 -- Revolute Joint/RConn1
  Rigid Transform2/RConn1 -- Revolute Joint/LConn1
  pendulum/RConn1 -- Tip/RConn1
  PS-Simulink Converter1/LConn1 -- Revolute Joint/RConn3
  pendulum/LConn1 -- Rigid Transform1/RConn1
  Rigid Transform2/LConn1 -- Spherical Solid/RConn1
  Revolute Joint/RConn2 -- PS-Simulink Converter3/LConn1
  Base/RConn1 -- Rigid Transform4/LConn1
  Rigid Transform4/RConn1 -- Rigid Transform3/LConn1
  Simulink-PS Converter/RConn1 -- Revolute Joint/LConn2
